simulink model "prb_4"  (R2020a)
settings: Solver=VariableStepAuto  StartTime=0.0  StopTime=10.0  RelTol=1e-3
settings Model: Creator=Riyansh  LastModifiedBy=Riyansh

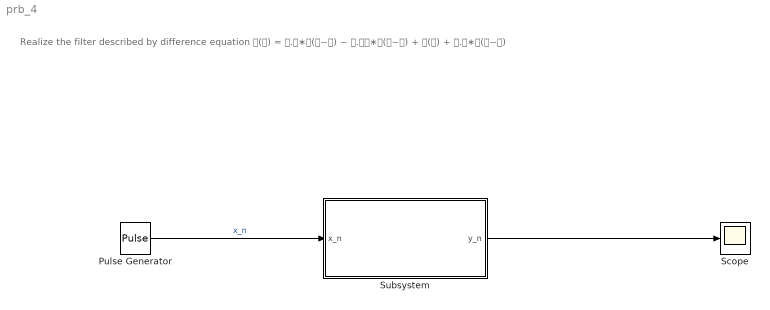
== system prb_4 ==
  note: Realize the filter described by difference equation 𝐲(𝐧) = 𝟎.𝟓∗𝐲(𝐧−𝟏) − 𝟎.𝟐𝟓∗𝐲(𝐧−𝟐) + 𝐱(𝐧) + 𝟎.𝟒∗𝐱(𝐧−𝟏)
  Pulse Generator : DiscretePulseGenerator  PulseType=Time based  Period=10  PulseWidth=5
  Scope : Scope
  Subsystem : Subsystem  TreatAsAtomicUnit=on
  wires:
  Pulse Generator/1 -> Subsystem/1(x_n)  "x_n"
  Subsystem/1(y_n) -> Scope/1

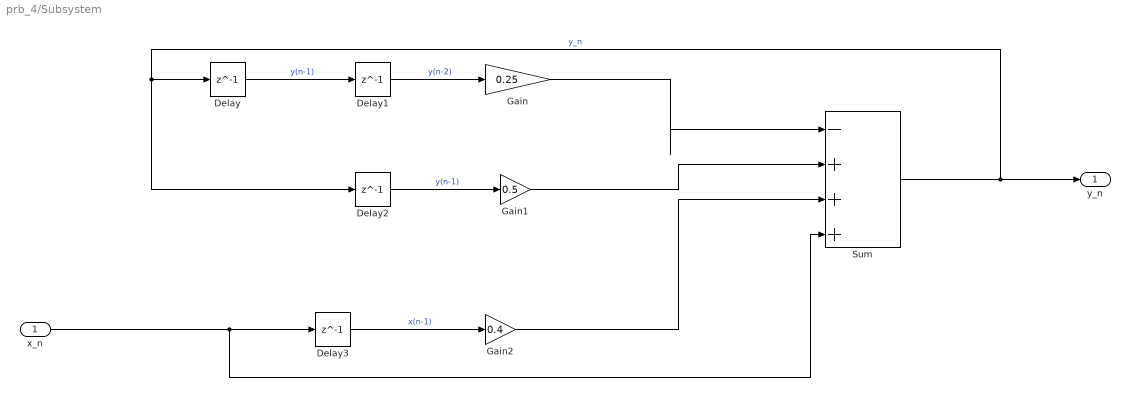
== system prb_4/Subsystem ==
  x_n : Inport
  Delay{,1..3} (4 alike) : Delay  DelayLength=1
  Gain : Gain  Gain=0.25
  Gain1 : Gain  Gain=0.5
  Gain2 : Gain  Gain=0.4
  Sum : Sum  Inputs=|-+++
  y_n : Outport
  wires:
  Gain2/1 -> Sum/3
  Delay2/1 -> Gain1/1  "y(n-1)"
  Sum/1 -> y_n/1, Delay/1, Delay2/1  "y_n"
  Delay1/1 -> Gain/1  "y(n-2)"
  Delay3/1 -> Gain2/1  "x(n-1)"
  Gain1/1 -> Sum/2
  Gain/1 -> Sum/1
  x_n/1 -> Sum/4, Delay3/1
  Delay/1 -> Delay1/1  "y(n-1)"
